simulink model "fullDiveHarness"  (R2026a)
settings: Solver=ode23t  StopTime=3900  MaxStep=0.1  RelTol=1e-4
undefined symbols (not defined in the file): ff_depths, ff_Vbcd, K_vff, Kd_b, Kp_b, profile_depth, profile_t, tau_lung, trim_max, V_bcd_max, V_lung_max, V_lung_min, V_mean, V_tidal, w_breath
libraries: simulink x2, fl_lib x2, simulink_extras x1
settings Model: Creator=grouleau  LastModifiedBy=grouleau

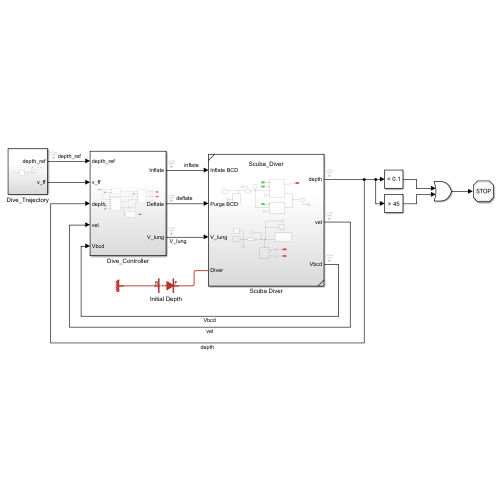
[thumbnail: Simulink's stored preview of the top-level diagram]
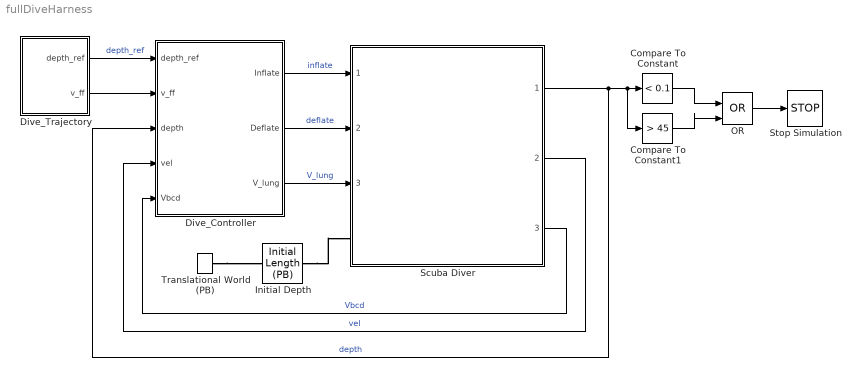
== system fullDiveHarness ==
  Compare To Constant : simulink/Logic and Bit Operations/Compare To Constant  relop=<  const=0.1  OutDataTypeStr=boolean
  Compare To Constant1 : simulink/Logic and Bit Operations/Compare To Constant  relop=>  const=45  OutDataTypeStr=boolean
  Dive_Controller : Subsystem
  Dive_Trajectory : Subsystem
  Initial Depth : fl_lib/Translational/Elements/Initial Length (PB)  length_specify=on  length_priority=High  length=0.5 m  length_nominal_specify=off  length_nominal_value=1  length_nominal_unit=m  f_specify=off  f_priority=None  f=0 N  f_nominal_specify=off  f_nominal_value=1  f_nominal_unit=N  v_rel_specify=off  v_rel_priority=None  v_rel=0 m/s  v_rel_nominal_specify=off  v_rel_nominal_value=1  v_rel_nominal_unit=m/s
  OR : Logic  Operator=OR  IconShape=distinctive  AllPortsSameDT=off  OutDataTypeStr=boolean
  Scuba Diver : Subsystem  ReferencedSubsystem=Scuba_Diver
  Stop Simulation : Stop
  Translational World (PB) : fl_lib/Translational/Elements/Translational World (PB)
  wires:
  Scuba Diver/2 -> Dive_Controller/4(vel)  "vel"
  Compare To Constant/1 -> OR/1
  OR/1 -> Stop Simulation/1
  Compare To Constant1/1 -> OR/2
  Scuba Diver/1 -> Compare To Constant1/1, Compare To Constant/1, Dive_Controller/3(depth)  "depth"
  Dive_Trajectory/1(depth_ref) -> Dive_Controller/1(depth_ref)  "depth_ref"
  Dive_Trajectory/2(v_ff) -> Dive_Controller/2(v_ff)
  Scuba Diver/3 -> Dive_Controller/5(Vbcd)  "Vbcd"
  Dive_Controller/1(Inflate) -> Scuba Diver/1  "inflate"
  Dive_Controller/2(Deflate) -> Scuba Diver/2  "deflate"
  Dive_Controller/3(V_lung) -> Scuba Diver/3  "V_lung"
  connections:
  Translational World (PB)/RConn1 -- Initial Depth/LConn1
  Initial Depth/RConn1 -- Scuba Diver/LConn1

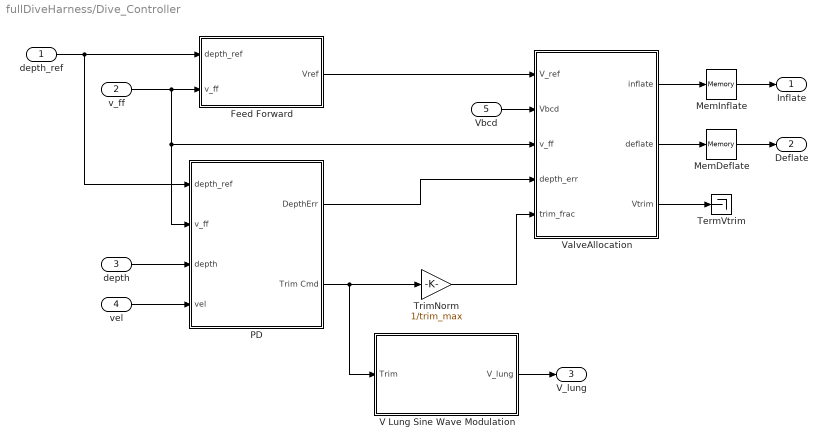
== system fullDiveHarness/Dive_Controller ==
  depth_ref : Inport
  v_ff : Inport  Port=2
  depth : Inport  Port=3
  vel : Inport  Port=4
  Vbcd : Inport  Port=5
  Feed Forward : Subsystem
  MemDeflate : Memory
  MemInflate : Memory
  PD : Subsystem
  TermVtrim : Terminator
  TrimNorm : Gain  Gain=1/trim_max
  V Lung Sine Wave Modulation : Subsystem
  ValveAllocation : Stateflow chart  TreatAsAtomicUnit=on
  Inflate : Outport
  Deflate : Outport  Port=2
  V_lung : Outport  Port=3
  wires:
  V Lung Sine Wave Modulation/1(V_lung) -> V_lung/1
  vel/1 -> PD/4(vel)
  depth/1 -> PD/3(depth)
  depth_ref/1 -> PD/1(depth_ref), Feed Forward/1(depth_ref)
  v_ff/1 -> PD/2(v_ff), ValveAllocation/3(v_ff), Feed Forward/2(v_ff)
  PD/2(Trim Cmd) -> TrimNorm/1, V Lung Sine Wave Modulation/1(Trim)
  MemInflate/1 -> Inflate/1
  MemDeflate/1 -> Deflate/1
  Feed Forward/1(Vref) -> ValveAllocation/1(V_ref)
  Vbcd/1 -> ValveAllocation/2(Vbcd)
  PD/1(DepthErr) -> ValveAllocation/4(depth_err)
  TrimNorm/1 -> ValveAllocation/5(trim_frac)
  ValveAllocation/1(inflate) -> MemInflate/1
  ValveAllocation/2(deflate) -> MemDeflate/1
  ValveAllocation/3(Vtrim) -> TermVtrim/1

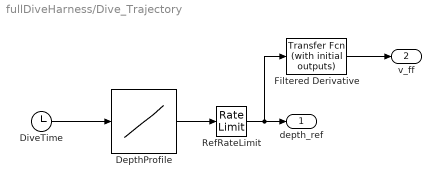
== system fullDiveHarness/Dive_Trajectory ==
  DepthProfile : Lookup_n-D  NumberOfTableDimensions=1  BreakpointsForDimension1=profile_t  Table=profile_depth  ExtrapMethod=Clip  InternalRulePriority=Speed  RndMeth=Simplest
  DiveTime : Clock
  Filtered Derivative : simulink_extras/Additional Linear/Transfer Fcn (with initial outputs)  N=[1 0]  D="[0.1  1]"  Y0=0.146  U0=0.5
  RefRateLimit : RateLimiter  RisingSlewLimit=0.3  FallingSlewLimit=-0.15
  depth_ref : Outport
  v_ff : Outport  Port=2
  wires:
  RefRateLimit/1 -> Filtered Derivative/1, depth_ref/1
  DiveTime/1 -> DepthProfile/1
  DepthProfile/1 -> RefRateLimit/1
  Filtered Derivative/1 -> v_ff/1

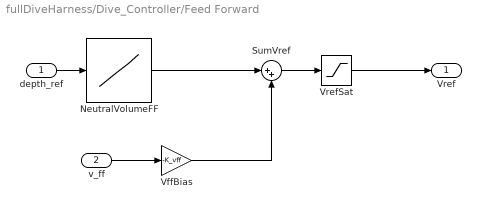
== system fullDiveHarness/Dive_Controller/Feed Forward ==
  depth_ref : Inport
  v_ff : Inport  Port=2
  NeutralVolumeFF : Lookup_n-D  NumberOfTableDimensions=1  BreakpointsForDimension1=ff_depths  Table=ff_Vbcd  ExtrapMethod=Clip  InternalRulePriority=Speed  RndMeth=Simplest
  SumVref : Sum  Inputs=|++
  VffBias : Gain  Gain=-K_vff
  VrefSat : Saturate  UpperLimit=V_bcd_max  LowerLimit=0
  Vref : Outport
  wires:
  VffBias/1 -> SumVref/2
  SumVref/1 -> VrefSat/1
  v_ff/1 -> VffBias/1
  NeutralVolumeFF/1 -> SumVref/1
  depth_ref/1 -> NeutralVolumeFF/1
  VrefSat/1 -> Vref/1

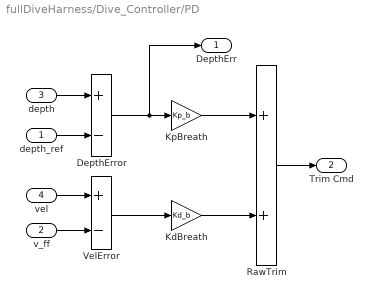
== system fullDiveHarness/Dive_Controller/PD ==
  depth_ref : Inport
  v_ff : Inport  Port=2
  depth : Inport  Port=3
  vel : Inport  Port=4
  DepthError : Sum  Inputs=+-
  KdBreath : Gain  Gain=Kd_b
  KpBreath : Gain  Gain=Kp_b
  RawTrim : Sum
  VelError : Sum  Inputs=+-
  DepthErr : Outport
  Trim Cmd : Outport  Port=2
  wires:
  KdBreath/1 -> RawTrim/2
  depth/1 -> DepthError/1
  vel/1 -> VelError/1
  v_ff/1 -> VelError/2
  VelError/1 -> KdBreath/1
  KpBreath/1 -> RawTrim/1
  depth_ref/1 -> DepthError/2
  DepthError/1 -> DepthErr/1, KpBreath/1
  RawTrim/1 -> Trim Cmd/1

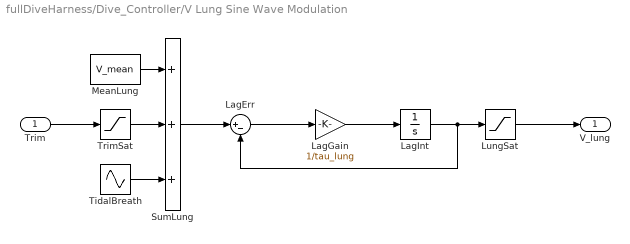
== system fullDiveHarness/Dive_Controller/V Lung Sine Wave Modulation ==
  Trim : Inport
  LagErr : Sum  Inputs=|+-
  LagGain : Gain  Gain=1/tau_lung
  LagInt : Integrator  InitialCondition=V_mean
  LungSat : Saturate  UpperLimit=V_lung_max  LowerLimit=V_lung_min
  MeanLung : Constant  Value=V_mean
  SumLung : Sum  Inputs=+++
  TidalBreath : Sin  Amplitude=V_tidal  Frequency=w_breath  SampleTime=0
  TrimSat : Saturate  UpperLimit=trim_max  LowerLimit=-trim_max
  V_lung : Outport
  wires:
  SumLung/1 -> LagErr/1
  TidalBreath/1 -> SumLung/3
  LagInt/1 -> LungSat/1, LagErr/2
  TrimSat/1 -> SumLung/2
  MeanLung/1 -> SumLung/1
  LagErr/1 -> LagGain/1
  LagGain/1 -> LagInt/1
  Trim/1 -> TrimSat/1
  LungSat/1 -> V_lung/1

== stateflow chart fullDiveHarness/Dive_Controller/ValveAllocation ==
  settings: updateMethod=DISCRETE  sampleTime=0.1
  state ValveLogic
    du:
    % low-pass the breathing trim so tidal oscillation cannot mask saturation
    trimF = trimF + (Ts/tau_f)*(trim_frac - trimF);
    state Hold
      en:
      % neutrally trimmed: valves stay shut, breathing does the fine control
      inflate = 0;
      deflate = 0;
    state Maneuvering
      du:
      % depth transition: track the feedforward bladder volume
      servo();
    state ReTrimBurst
      du:
      % short valve window to re-center the breathing trim
      servo();
    (default) -> Hold
    Maneuvering -> Hold : [abs(v_ff) < 1e-4 && abs(depth_err) <= 1]
    Hold -> Maneuvering [order 1] : [abs(v_ff) >= 1e-4 || abs(depth_err) > 1]
    ReTrimBurst -> Hold : [after(burst_t, sec)]
    Hold -> ReTrimBurst [order 2] : [duration(abs(trimF) > sat_lvl) >= sat_t]{Vtrim = Vtrim + sign(trimF)*step_V;}
  (default) -> ValveLogic
  data: V_ref input double; Vbcd input double; v_ff input double; depth_err input double; trim_frac input double; inflate output double =0; deflate output double =0; Vtrim output double =0; trimF local double =0; db constant double =0.15e-3; k_inf constant double =300; inf_max constant double =0.6; k_def constant double =300; sat_lvl constant double =0.6; sat_t constant double =15; step_V constant double =0.2e-3; burst_t constant double =5; tau_f constant double =5; Ts constant double =0.1
  function servo:
    | function servo
    | % Deadband volume servo on the BCD bladder.
    | % Acts on the volume error against the feedforward + slow-trim reference.
    | e = (V_ref + Vtrim) - Vbcd;
    | inflate = 0;
    | deflate = 0;
    | if e > db
    |     inflate = min(k_inf*(e - db), inf_max);
    | elseif e < -db
    |     deflate = min(k_def*(-e - db), 1);
    | end
    | end
